simulink model "BPSK"  (R2021a)
settings: Solver=VariableStepAuto  StartTime=0.0  StopTime=10.0  RelTol=1e-3
libraries: commchan3 x2, commdigbbndpm3 x2, commsink2 x2, commdigbbndfm2 x2, commsrccod2 x1, commrandsrc3 x1, dspsigops x1, dspquant2 x1
settings Model: Creator=Bharat Gunhalkar  LastModifiedBy=Bharat Gunhalkar

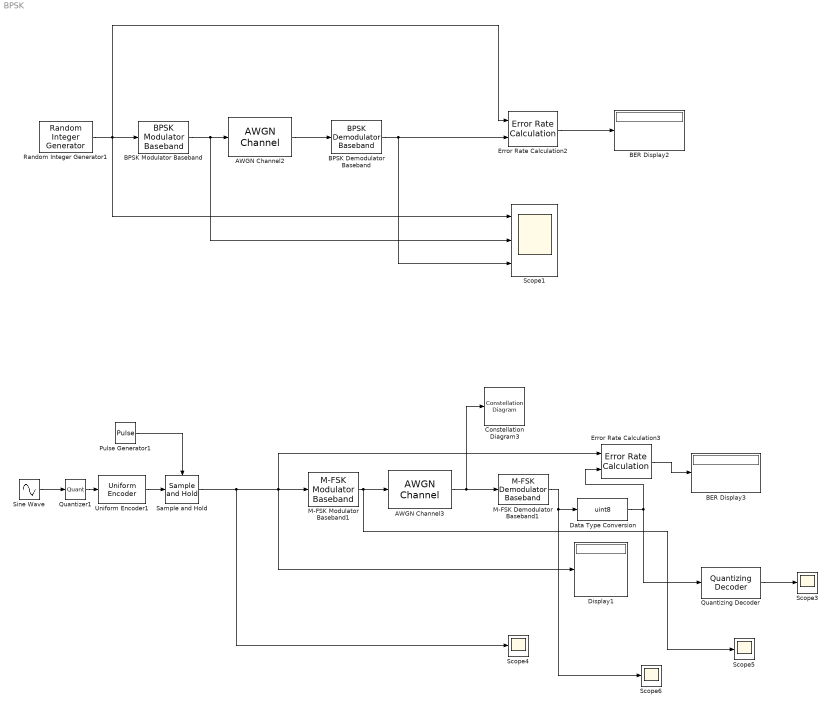
== system BPSK ==
  AWGN Channel2 : commchan3/AWGN Channel  InputProcessing=Columns as channels (frame based)  seed=67  noiseMode="Signal to noise ratio  (Eb/No)"  EbNodB=1  EsNodB=10  SNRdB=10  bitsPerSym=1  Ps=1  Tsym=1  variance=1
  AWGN Channel3 : commchan3/AWGN Channel  InputProcessing=Columns as channels (frame based)  seed=67  noiseMode="Signal to noise ratio  (Eb/No)"  EbNodB=100  EsNodB=10  SNRdB=10  bitsPerSym=1  Ps=1  Tsym=1  variance=1
  BER Display2 : Display
  BER Display3 : Display
  BPSK Demodulator Baseband : commdigbbndpm3/BPSK Demodulator Baseband  DecType=Hard decision  VarSource=Dialog  Variance=1  Ph=0  outDtype=Inherit via internal rule  derotateFactorWordLen=16  derotateFactorDataTypeStr=Inherit: Same word length as input  derotateFactorLastDataTypeStr=Inherit: Same word length as input
  BPSK Modulator Baseband : commdigbbndpm3/BPSK Modulator Baseband  Ph=0  outDtype=double  outWordLen=16  outUDDataType=sfix(16)  outFracLenMode=Best precision  outFracLen=15  outDataTypeStr=double  outLastDataTypeStr=double
  Constellation Diagram3 : ConstellationDiagram
  Data Type Conversion : DataTypeConversion  OutDataTypeStr=uint8
  Display1 : Display
  Error Rate Calculation2 : commsink2/Error Rate Calculation  N=0  st_delay=0  cp_mode=Entire frame  subframe=[]  PMode=Port  WsName=ErrorVec  RsMode2=off  stop=off  numErr=100  maxBits=1e6
  Error Rate Calculation3 : commsink2/Error Rate Calculation  N=0  st_delay=0  cp_mode=Entire frame  subframe=[]  PMode=Port  WsName=ErrorVec  RsMode2=off  stop=off  numErr=100  maxBits=1e6
  M-FSK Demodulator Baseband1 : commdigbbndfm2/M-FSK Demodulator Baseband  M=8  OutType=Integer  Dec=Gray  freqSep=6  numSamp=17  RateOptions=Enforce single-rate processing  outDataType=double
      settings: SourceProductBaseCode=CM
  M-FSK Modulator Baseband1 : commdigbbndfm2/M-FSK Modulator Baseband  M=8  InType=Integer  Enc=Gray  freqSep=6  phaseType=Continuous  numSamp=17  RateOptions=Enforce single-rate processing  outDataType=double
  Pulse Generator1 : DiscretePulseGenerator  SampleTime=0.001
  Quantizer1 : Quantizer  QuantizationInterval=.333
  Quantizing Decoder : commsrccod2/Quantizing Decoder  codebook=[-.825 -.5 0, .5 .825]  QuDType=double
      settings: SourceProductBaseCode=CM
  Random Integer Generator1 : commrandsrc3/Random Integer Generator  SetSize=2  SeedSource=Auto  Seed=0  SampleTime=0.1  SamplesPerFrame=1  OutputDataType=double  SimulateUsing=Interpreted execution
  Sample and Hold : dspsigops/Sample and Hold  trig=Rising edge  initCond=0  latchinput=off
  Scope1 : Scope  NumInputPorts=3
  Scope{3..6} (4 alike) : Scope
  Sine Wave : Sin  Amplitude=5  Frequency=2*pi  SampleTime=0.001
  Uniform Encoder1 : dspquant2/Uniform Encoder  peak=1  bits=3  otype=Unsigned integer
  wires:
  BPSK Modulator Baseband/1 -> Scope1/2, AWGN Channel2/1
  Random Integer Generator1/1 -> Scope1/1, BPSK Modulator Baseband/1, Error Rate Calculation2/1
  BPSK Demodulator Baseband/1 -> Error Rate Calculation2/2, Scope1/3
  Error Rate Calculation2/1 -> BER Display2/1
  AWGN Channel2/1 -> BPSK Demodulator Baseband/1
  Sine Wave/1 -> Quantizer1/1
  Quantizer1/1 -> Uniform Encoder1/1
  M-FSK Modulator Baseband1/1 -> Scope5/1, AWGN Channel3/1
  M-FSK Demodulator Baseband1/1 -> Scope6/1, Data Type Conversion/1
  AWGN Channel3/1 -> M-FSK Demodulator Baseband1/1, Constellation Diagram3/1
  Error Rate Calculation3/1 -> BER Display3/1
  Data Type Conversion/1 -> Quantizing Decoder/1, Error Rate Calculation3/2
  Pulse Generator1/1 -> Sample and Hold/Trigger
  Uniform Encoder1/1 -> Sample and Hold/1
  Quantizing Decoder/1 -> Scope3/1
  Sample and Hold/1 -> Scope4/1, Display1/1, Error Rate Calculation3/1, M-FSK Modulator Baseband1/1
